simulink model "comp_modelR2015a"  (R2015a)
settings: Solver=ode3  SolverMode=SingleTasking  StartTime=0.0  StopTime=1  FixedStep=0.01  RelTol=1e-3
values from neighbouring files (symbols this model uses):
  A = [0 1 0 0; -K_m/M 0 K_m/M 0; 0 0 0 1; K_m/M 0 -K_m/M 0]    [desafio1.m]
  B = [0 0; 1/M 0; 0 0; 0 1/M]    [desafio1.m]
  C = [1 0 0 0; 0 0 1 0]    [desafio1.m]
  F = -lqr(A,B,eye(4),eye(2),0)    [desafio1.m]
  K = lqr(A.',C.',eye(4),eye(2),0)'    [desafio1.m]
  r = [1; 1]    [desafio1.m]
  x0 = [0; 0; 0; 0]    [desafio1.m]
settings Model: CovMetricSettings=dwe  CovHtmlReporting=off  covSaveCumulativeToWorkspaceVar=off  CovSaveSingleToWorkspaceVar=off  CovExternalEMLEnable=on  Creator=Murillo  LastModifiedBy=vinic
settings DataIOCC: LimitDataPoints=off  SaveFormat=Dataset  ReturnWorkspaceOutputs=on
settings DebuggingCC: SFUnexpectedBacktrackingDiag=error  SFNoUnconditionalDefaultTransitionDiag=error
settings HardwareCC: ProdBitPerPointer=64  ProdLargestAtomicFloat=Float  ProdIntDivRoundTo=Zero  ProdEndianess=LittleEndian  ProdHWDeviceType=Specified
settings ModelReferenceCC: PropagateSignalLabelsOutOfModel=on
settings SFSimCC: SimUseLocalCustomCode=on
settings RTWCC: RTWUseLocalCustomCode=on
settings GRTTargetCC: TargetLangStandard=C99 (ISO)

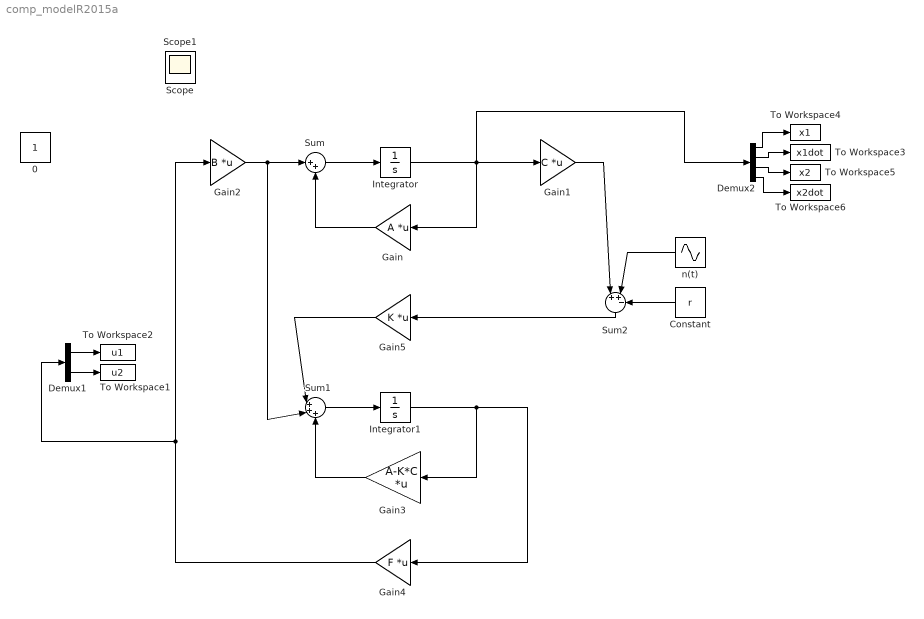
== system comp_modelR2015a ==
  Constant : Constant  Value=r  VectorParams1D=off
  Demux1 : Demux  Outputs=2
  Demux2 : Demux
  Gain : Gain  Gain=A  Multiplication=Matrix(K*u)
  Gain1 : Gain  Gain=C  Multiplication=Matrix(K*u)
  Gain2 : Gain  Gain=B  Multiplication=Matrix(K*u)
  Gain3 : Gain  Gain=A-K*C  Multiplication=Matrix(K*u)
  Gain4 : Gain  Gain=F  Multiplication=Matrix(K*u)
  Gain5 : Gain  Gain=K  Multiplication=Matrix(K*u)
  Integrator : Integrator  InitialCondition=x0
  Integrator1 : Integrator
  Sum : Sum  Inputs=|++
  Sum1 : Sum  Inputs=|+++
  Sum2 : Sum  Inputs=|++-
  To Workspace1 : ToWorkspace  VariableName=u2  SampleTime=-1
      settings: Save2DSignal=2-D array (concatenate along first dimension)
  To Workspace2 : ToWorkspace  VariableName=u1  SampleTime=-1
      settings: Save2DSignal=2-D array (concatenate along first dimension)
  To Workspace3 : ToWorkspace  VariableName=x1dot  SampleTime=-1
      settings: Save2DSignal=2-D array (concatenate along first dimension)
  To Workspace4 : ToWorkspace  VariableName=x1  SampleTime=-1
      settings: Save2DSignal=2-D array (concatenate along first dimension)
  To Workspace5 : ToWorkspace  VariableName=x2  SampleTime=-1
      settings: Save2DSignal=2-D array (concatenate along first dimension)
  To Workspace6 : ToWorkspace  VariableName=x2dot  SampleTime=-1
      settings: Save2DSignal=2-D array (concatenate along first dimension)
  n(t) : Sin  Amplitude=0.05  Frequency=20  SampleTime=0
  0 : Constant  IOType=siggen
  Scope : Scope
      settings: TimeRange=auto  MaxDataPoints=5000  SaveToWorkspace=off  SaveName=ScopeData  YMin=-10.00000  YMax=10.00000  SampleTime=-1
  Scope1 : Scope
      settings: TimeRange=auto  MaxDataPoints=5000  SaveToWorkspace=off  YMin=-10.00000  YMax=10.00000  SampleTime=-1
  wires:
  Sum/1 -> Integrator/1
  Gain/1 -> Sum/2
  Gain2/1 -> Sum1/2, Sum/1
  Sum1/1 -> Integrator1/1
  Integrator1/1 -> Gain3/1, Gain4/1
  Gain3/1 -> Sum1/3
  Gain4/1 -> Demux1/1, Gain2/1
  Gain1/1 -> Sum2/1
  Sum2/1 -> Gain5/1
  Gain5/1 -> Sum1/1
  Constant/1 -> Sum2/3
  Integrator/1 -> Gain/1, Demux2/1, Gain1/1
  Demux2/2 -> To Workspace3/1
  Demux2/4 -> To Workspace6/1
  Demux2/1 -> To Workspace4/1
  Demux2/3 -> To Workspace5/1
  Demux1/1 -> To Workspace2/1
  Demux1/2 -> To Workspace1/1
  n(t)/1 -> Sum2/2
